simulink model "test66"  (R2015a)
settings: Solver=ode4  StartTime=0.0  StopTime=10  FixedStep=0.001  RelTol=1e-3
values from neighbouring files (symbols this model uses):
  A = [[   0      1         0         0         0         0] ... (first row only)    [test2.m]    (also in test3.m = [[   0      0         0         1         0         0]; test4.m = [[   0      0         0         1         0         0]; test5.m = [[zeros(2,2) eye(2)];[dg zeros(2,2)]])
  Ac = A - B*K + L*C    [test3.m]    (also in test4.m; test5.m)
  B = [0 22.07202 0 -151.371141 0 -56.32414]'    [test2.m]    (also in test3.m = [0 0 0 -0.6070 1.4984 -0.2839]'; test4.m = [0 0 0 -0.6070 1.4984 -0.2839]'; test5.m = [[zeros(2,1)]; [di*h]])
  Bc = -L    [test3.m]    (also in test4.m; test5.m)
  C = [1 0 0 0 0 0]    [test2.m]    (also in test3.m; test4.m; test5.m = [1 0 0 0])
  Cc = K    [test3.m]    (also in test4.m; test5.m)
  D = 0    [test2.m]    (also in test3.m; test4.m; test5.m)
  d1 = m0 + m1 + m2    (= 2.75)    [test3.m]    (also in test4.m; test5.m = 0.00498784618394)
  d2 = (m1/2 + m2) * l1    (= 0.5)    [test3.m]    (also in test4.m; test5.m = 0.00670234055869)
  d3 = m2 * l2/2    (= 0.28125)    [test3.m]    (also in test4.m; test5.m = 0.00902586221044)
  Dc = 0    [test3.m]    (also in test4.m; test5.m)
  f1 = (m1/2 + m2) * l1 * g    (= 4.9)    [test3.m]    (also in test4.m; test5.m = 0.66350669926)
  f2 = m2 * l2 *g/2    (= 2.75625)    [test3.m]    (also in test4.m; test5.m = 0.891162386564)
  r = 0    [test2.m]    (also in test3.m; test4.m; test5.m)
settings Model: Creator=joseg  LastModifiedBy=joseg

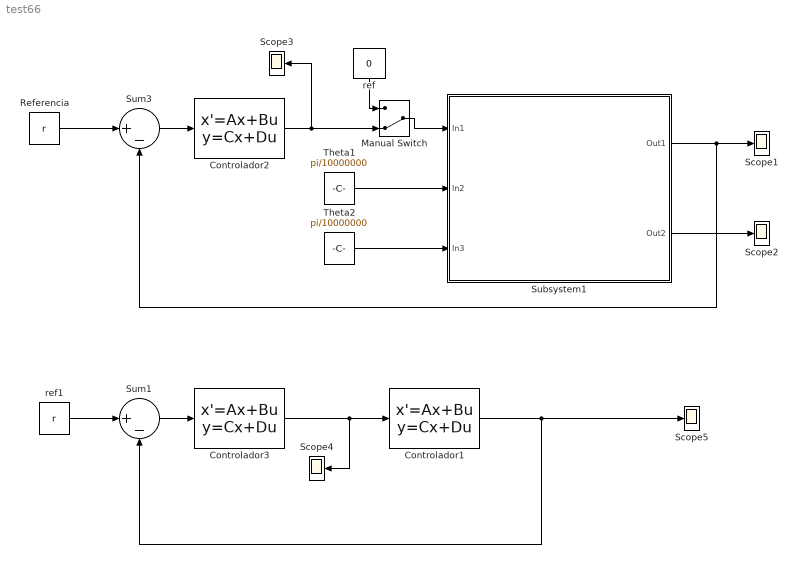
== system test66 ==
  Controlador1 : StateSpace  A=A  B=B  C=C  D=D  X0=[0;0;0;0]
  Controlador2 : StateSpace  A=Ac  B=Bc  C=Cc  D=Dc  X0=[0;0;0;0]
  Controlador3 : StateSpace  A=Ac  B=Bc  C=Cc  D=Dc  X0=[pi/10000000;pi/10000000;0;0]
  Manual Switch : ManualSwitch  CurrentSetting=0
  Referencia : Constant  Value=r
  Scope{1..5} (5 alike) : Scope
      Scope1 settings: TimeRange=14.3  YMin=-3.5e+21  YMax=0
      Scope2 settings: TimeRange=14.3  YMin=-3.5e+21  YMax=0
      Scope3 settings: TimeRange=14.3  YMin=-3.5e+21  YMax=0  SaveName=ScopeData2
      Scope4 settings: TimeRange=14.3  YMin=-3.5e+21  YMax=0  SaveName=ScopeData4
      Scope5 settings: TimeRange=14.3  YMin=-3.5e+21  YMax=0  SaveName=ScopeData3
  Subsystem1 : Subsystem
  Sum1 : Sum  Inputs=|+-
  Sum3 : Sum  Inputs=|+-
  Theta1 : Constant  Value=pi/10000000
  Theta2 : Constant  Value=pi/10000000
  ref : Constant  Value=0
  ref1 : Constant  Value=r
  wires:
  Theta1/1 -> Subsystem1/2(In2)
  Theta2/1 -> Subsystem1/3(In3)
  Sum3/1 -> Controlador2/1
  Subsystem1/1(Out1) -> Sum3/2, Scope1/1
  Referencia/1 -> Sum3/1
  Controlador2/1 -> Scope3/1, Manual Switch/2
  Manual Switch/1 -> Subsystem1/1(In1)
  ref/1 -> Manual Switch/1
  Controlador1/1 -> Scope5/1, Sum1/2
  Controlador3/1 -> Scope4/1, Controlador1/1
  Sum1/1 -> Controlador3/1
  ref1/1 -> Sum1/1
  Subsystem1/2(Out2) -> Scope2/1

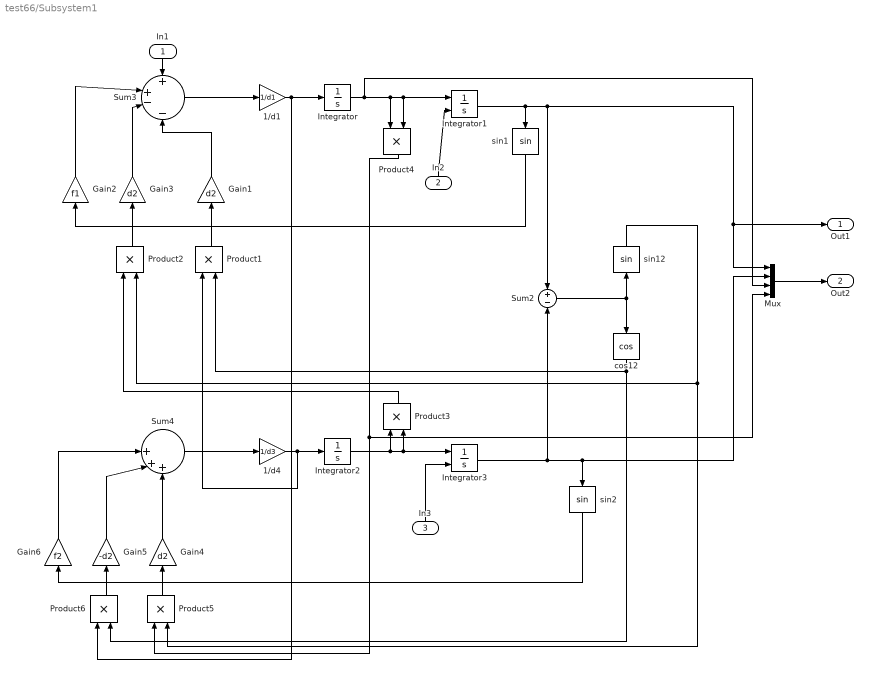
== system test66/Subsystem1 ==
  In1 : Inport
  In2 : Inport  Port=2
  In3 : Inport  Port=3
  1/d1 : Gain  Gain=1/d1
  1/d4 : Gain  Gain=1/d3
  Gain1 : Gain  Gain=d2
  Gain2 : Gain  Gain=f1
  Gain3 : Gain  Gain=d2
  Gain4 : Gain  Gain=d2
  Gain5 : Gain  Gain=-d2
  Gain6 : Gain  Gain=f2
  Integrator : Integrator
  Integrator1 : Integrator  InitialConditionSource=external
  Integrator2 : Integrator
  Integrator3 : Integrator  InitialConditionSource=external
  Mux : Mux
  Product{1..6} (6 alike) : Product
  Sum2 : Sum  Inputs=+|-
  Sum3 : Sum  Inputs=+|+-|-
  Sum4 : Sum  Inputs=||+++
  cos12 : Trigonometry  Operator=cos
  sin1 : Trigonometry
  sin12 : Trigonometry
  sin2 : Trigonometry
  Out1 : Outport
  Out2 : Outport  Port=2
  wires:
  sin12/1 -> Product5/2, Product2/2
  Integrator2/1 -> Integrator3/1, Product3/2, Product3/1
  Product3/1 -> Product2/1
  Product6/1 -> Gain5/1
  Integrator/1 -> Mux/3, Product4/1, Product4/2, Integrator1/1
  Product5/1 -> Gain4/1
  Gain5/1 -> Sum4/2
  sin1/1 -> Gain2/1
  Gain4/1 -> Sum4/3
  cos12/1 -> Product6/2, Product1/2
  1/d4/1 -> Integrator2/1, Product1/1
  Product4/1 -> Product5/1, Mux/4
  Product2/1 -> Gain3/1
  In1/1 -> Sum3/1
  Gain6/1 -> Sum4/1
  Product1/1 -> Gain1/1
  Gain2/1 -> Sum3/2
  Gain1/1 -> Sum3/4
  sin2/1 -> Gain6/1
  Sum4/1 -> 1/d4/1
  1/d1/1 -> Integrator/1, Product6/1
  Sum3/1 -> 1/d1/1
  Integrator3/1 -> sin2/1, Mux/2, Sum2/2
  Sum2/1 -> cos12/1, sin12/1
  Integrator1/1 -> sin1/1, Sum2/1, Mux/1, Out1/1
  Gain3/1 -> Sum3/3
  In2/1 -> Integrator1/2
  In3/1 -> Integrator3/2
  Mux/1 -> Out2/1
